simulink model "mod02"  (R2012b)
settings: Solver=ode3  StartTime=0.0  StopTime=100  FixedStep=0.001  RelTol=1e-3
settings Model: Creator=NTB  LastModifiedBy=NTB

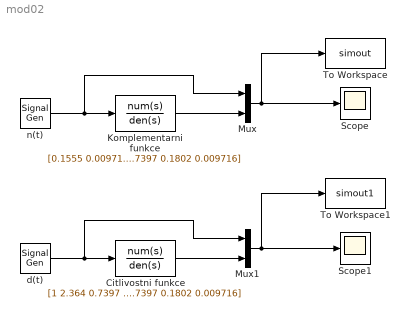
== system mod02 ==
  Citlivostni funkce : TransferFcn  Numerator=[1 2.364 0.7397 0.02479 0]  Denominator=[1 2.364 0.7397 0.1802 0.009716]
  Komplementarni funkce : TransferFcn  Numerator=[0.1555 0.00971]  Denominator=[1 2.364 0.7397 0.1802 0.009716]
  Mux : Mux  Inputs=2
  Mux1 : Mux  Inputs=2
  Scope : Scope
      settings: YMin=-1.75  YMax=1.75
  Scope1 : Scope
  To Workspace : ToWorkspace  VariableName=simout  SampleTime=-1  SaveFormat=Timeseries
  To Workspace1 : ToWorkspace  VariableName=simout1  SampleTime=-1  SaveFormat=Timeseries
  d(t) : SignalGenerator  Frequency=0.322  Units=rad/sec
  n(t) : SignalGenerator  Frequency=0.194  Units=rad/sec
  wires:
  Mux/1 -> To Workspace/1, Scope/1
  Komplementarni funkce/1 -> Mux/2
  n(t)/1 -> Mux/1, Komplementarni funkce/1
  Mux1/1 -> To Workspace1/1, Scope1/1
  Citlivostni funkce/1 -> Mux1/2
  d(t)/1 -> Mux1/1, Citlivostni funkce/1
